simulink model "sltank2"  (R2018b)
settings: Solver=ode23  StartTime=0  StopTime=10000  MaxStep=0.2  RelTol=1e-3  AbsTol=1e-6
PreLoadFcn:
  | tank2=readfis('tank2');
libraries: fuzblock x1, simulink x1
CloseFcn:
  | clear tank2
settings Model: FPTRunName=Active  ExtModeTrigMode=oneshot  ExtModeArmWhenConnect=off  ExtModeAutoUpdateStatusClock=off  Creator=The MathWorks, Inc.  LastModifiedBy=The MathWorks, Inc.
settings SolverCC: AutoScaleAbsTol=off
settings DataIOCC: SaveFormat=Array  SaveOutput=off  SaveTime=off
settings OptimizationCC: BlockReduction=off  BooleanDataType=off  ExpressionDepthLimit=2147483647  InitFltsAndDblsToZero=on  LifeSpan=inf
settings DebuggingCC: SaveWithParameterizedLinksMsg=none  UnderspecifiedInitializationDetection=Classic  MergeDetectMultiDrivingBlocksExec=none  SignalResolutionControl=TryResolveAllWithWarning  MultiTaskDSMMsg=warning  MultiTaskCondExecSysMsg=none  FcnCallInpInsideContextMsg=warning  StateNameClashWarn=warning  LibraryContextMissingDiagnostic=none  SFUnexpectedBacktrackingDiag=warning  SFNoUnconditionalDefaultTransitionDiag=warning  SFExecutionAtInitializationDiag=none
settings HardwareCC: ProdBitPerPointer=32  ProdBitPerSizeT=32  ProdBitPerPtrDiffT=32  ProdLargestAtomicFloat=None  ProdIntDivRoundTo=Undefined  ProdEndianess=Unspecified  ProdWordSize=32  ProdHWDeviceType=32-bit Generic  TargetUnknown=on
settings ModelReferenceCC: PropagateSignalLabelsOutOfModel=off
settings SFSimCC: SimUseLocalCustomCode=off
settings RTWCC: RTWUseLocalCustomCode=off
settings CodeAppCC: StateflowObjectComments=on
settings GRTTargetCC: TargetFcnLib=ansi_tfl_tmw.mat  TargetLangStandard=C89/C90 (ANSI)  GeneratePreprocessorConditionals=Disable all  CombineOutputUpdateFcns=off  GRTInterface=on
settings ConfigComp: CovMetricSettings=dw  CovHtmlReporting=on  CovSaveCumulativeToWorkspaceVar=on  CovSaveSingleToWorkspaceVar=on  CovExternalEMLEnable=off

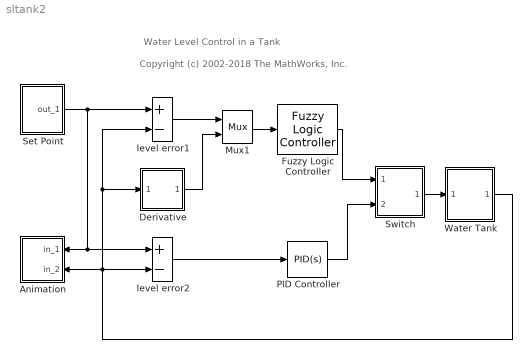
== system sltank2 ==
  note: Copyright (c) 2002-2018 The MathWorks, Inc.
  note: Water Level Control in a Tank
  Animation : Subsystem
  Derivative : Subsystem
  Fuzzy Logic Controller : fuzblock/Fuzzy Logic  Controller  FIS=tank2  OutputSampleNumber=101  DataType=double  FuzzifiedInputs=off  RuleFiringStrengths=off  RuleOutputs=off  AggregatedOutputs=off  SimulateUsing=Interpreted execution  OutOfRangeInputValueMessage=warning  NoRuleFiredMessage=warning  EmptyOutputFuzzySetMessage=warning
  Mux1 : Mux  Inputs=2
  PID Controller : simulink/Continuous/PID Controller  Controller=PID  Form=Parallel  TimeDomain=Continuous-time  SampleTime=1  IntegratorMethod=Forward Euler  FilterMethod=Forward Euler  ControllerParametersSource=internal  P=2  I=0  D=1  UseFilter=on  N=100  TunerSelectOption=Transfer Function Based (PID Tuner App)  InitialConditionSource=internal  InitialConditionForIntegrator=0  InitialConditionForFilter=0  DifferentiatorICPrevScaledInput=0  ExternalReset=none  TrackingMode=off  Kt=1  LimitOutput=off  UpperSaturationLimit=inf  LowerSaturationLimit=-inf  LinearizeAsGain=off  AntiWindupMode=none  Kb=1  POutMin=[]  POutMax=[]  IOutMin=[]  IOutMax=[]  DOutMin=[]  DOutMax=[]  NOutMin=[]  NOutMax=[]  SumOutMin=[]  SumOutMax=[]  SaturationOutMin=[]  SaturationOutMax=[]  PParamMin=[]  PParamMax=[]  IParamMin=[]  IParamMax=[]  DParamMin=[]  DParamMax=[]  NParamMin=[]  NParamMax=[]  KbParamMin=[]  KbParamMax=[]  KtParamMin=[]  KtParamMax=[]  KbOutMin=[]  KbOutMax=[]  KtOutMin=[]  KtOutMax=[]  IntegratorOutMin=[]  IntegratorOutMax=[]  FilterOutMin=[]  FilterOutMax=[]  SumI1OutMin=[]  SumI1OutMax=[]  SumI2OutMin=[]  SumI2OutMax=[]  SumI3OutMin=[]  SumI3OutMax=[]  SumI4OutMin=[]  SumI4OutMax=[]  SumDOutMin=[]  SumDOutMax=[]  DifferentiatorOutMin=[]  DifferentiatorOutMax=[]  FilterDiffOutCoefMin=[]  FilterDiffOutCoefMax=[]  ReciprocalOutMin=[]  ReciprocalOutMax=[]  SumDenOutMin=[]  SumDenOutMax=[]  SumNumOutMin=[]  SumNumOutMax=[]  DivideOutMin=[]  DivideOutMax=[]  IntegratorContinuousStateAttributes=''  IntegratorStateMustResolveToSignalObject=off  IntegratorRTWStateStorageClass=Auto  FilterContinuousStateAttributes=''  FilterStateMustResolveToSignalObject=off  FilterRTWStateStorageClass=Auto  ParallelPVariant=InternalParameters  IdealPVariant=Disabled  IVariant=InternalParameters  DVariant=InternalParameters  IntegratorVariant=Continuous  SatVariant=Disabled  AWVariant=Passthrough  PCopyVariant=Disabled  TRVariant=Disabled  FdbkBlocksVariant=Forward  IdealPFdbkVariant=Disabled  SatFdbkVariant=Disabled  DerivativeFilterVariant=ContFilter  NVariant=InternalParameters  NCopyVariant=Disabled  FilterICVariant=InternalICsFilter  IntegratorICVariant=InternalICs  ExternalResetVariant=Disabled  TRSumVariant=Passthrough  SumFdbkVariant=Disabled  SumVariant=Sum_PID
  Set Point : Subsystem
  Switch : Subsystem
  Water Tank : Subsystem
  level error1 : Sum  Inputs=+-  SaturateOnIntegerOverflow=on  InputSameDT=on  OutDataTypeStr=Inherit: Same as first input
  level error2 : Sum  Inputs=+-  SaturateOnIntegerOverflow=on  InputSameDT=on  OutDataTypeStr=Inherit: Same as first input
  wires:
  Water Tank/1(out_1) -> Derivative/1(in_1), level error1/2, Animation/2(in_2), level error2/2
  level error2/1 -> PID Controller/1
  Derivative/1(out_1) -> Mux1/2
  Set Point/1(out_1) -> level error2/1, Animation/1(in_1), level error1/1
  PID Controller/1 -> Switch/2(in_2)
  Fuzzy Logic Controller/1 -> Switch/1(in_1)
  Switch/1(out_1) -> Water Tank/1(in_1)
  level error1/1 -> Mux1/1
  Mux1/1 -> Fuzzy Logic Controller/1

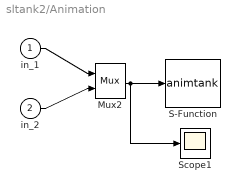
== system sltank2/Animation ==
  in_1 : Inport
  in_2 : Inport  Port=2
  Mux2 : Mux  Inputs=2
  S-Function : S-Function  FunctionName=animtank  Parameters=1  SFunctionDeploymentMode=off  EnableBusSupport=off
  Scope1 : Scope
  wires:
  in_2/1 -> Mux2/2
  in_1/1 -> Mux2/1
  Mux2/1 -> S-Function/1, Scope1/1

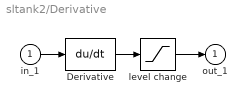
== system sltank2/Derivative ==
  in_1 : Inport
  Derivative : Derivative
  level change : Saturate  UpperLimit=0.1  LowerLimit=-0.1
  out_1 : Outport
  wires:
  in_1/1 -> Derivative/1
  level change/1 -> out_1/1
  Derivative/1 -> level change/1

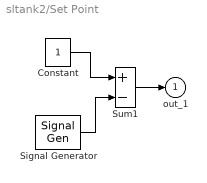
== system sltank2/Set Point ==
  Constant : Constant
  Signal Generator : SignalGenerator  WaveForm=square  Amplitude=0.500000  Frequency=0.250000  Units=rad/sec
  Sum1 : Sum  Inputs=+-  SaturateOnIntegerOverflow=on  InputSameDT=on  OutDataTypeStr=Inherit: Same as first input
  out_1 : Outport
  wires:
  Sum1/1 -> out_1/1
  Constant/1 -> Sum1/1
  Signal Generator/1 -> Sum1/2

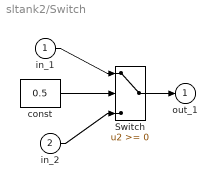
== system sltank2/Switch ==
  in_1 : Inport
  in_2 : Inport  Port=2
  Switch : Switch  SaturateOnIntegerOverflow=on  InputSameDT=on
  const : Constant  Value=0.5
  out_1 : Outport
  wires:
  in_2/1 -> Switch/3
  Switch/1 -> out_1/1
  in_1/1 -> Switch/1
  const/1 -> Switch/2

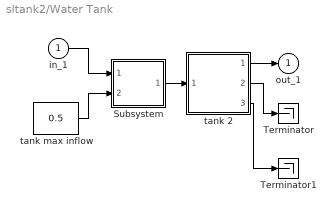
== system sltank2/Water Tank ==
  in_1 : Inport
  Subsystem : Subsystem  mask(Valve){InitialPosition=0}
      mask prompts: InitialPosition "Initial position [0=closed 1=open]:"
      mask help: Valve
      mask Display: disp('VALVE')
  Terminator : Terminator
  Terminator1 : Terminator
  tank 2 : Subsystem  mask(Water tank){ht=2, area=1, outletArea=0.05, overflowLimit=0, initialHt=0.5}
      mask prompts: ht "Height of tank (m):"; area "Bottom area (m^2):"; outletArea "Out pipe crossection (m^2):"; overflowLimit "Overflow sensor distance from top (m):"; initialHt "Initial level height (m):"
      mask help: Cylindrical water tank with overflow signal
      mask Display: disp('WATER\nTANK')
  tank max inflow : Constant  Value=0.5
  out_1 : Outport
  wires:
  Subsystem/1(out flow) -> tank 2/1(flow in)
  tank max inflow/1 -> Subsystem/2(source flow)
  tank 2/1(water level) -> out_1/1
  in_1/1 -> Subsystem/1(control)
  tank 2/2(flow out) -> Terminator/1
  tank 2/3(overflow flag) -> Terminator1/1

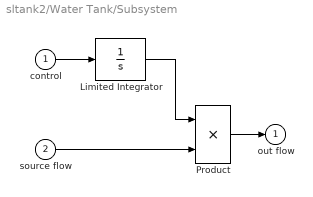
== system sltank2/Water Tank/Subsystem ==
  control : Inport
  source flow : Inport  Port=2
  Limited Integrator : Integrator  InitialCondition=InitialPosition  LimitOutput=on  UpperSaturationLimit=1  LowerSaturationLimit=0
  Product : Product  SaturateOnIntegerOverflow=on  RndMeth=Zero  InputSameDT=on  OutDataTypeStr=Inherit: Same as first input
  out flow : Outport
  wires:
  source flow/1 -> Product/2
  Product/1 -> out flow/1
  control/1 -> Limited Integrator/1
  Limited Integrator/1 -> Product/1

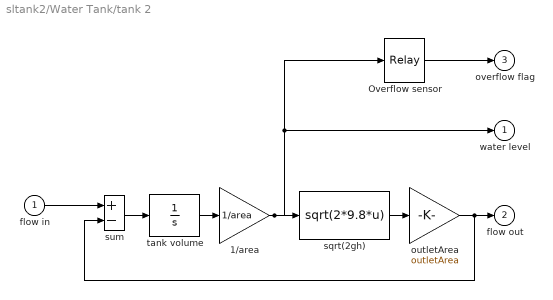
== system sltank2/Water Tank/tank 2 ==
  flow in : Inport
  1/area : Gain  Gain=1/area  SaturateOnIntegerOverflow=on  OutDataTypeStr=Inherit: Same as input  ParamDataTypeStr=Inherit: Same as input
  Overflow sensor : Relay  OnSwitchValue=ht - overflowLimit  OffSwitchValue=ht - overflowLimit
  outletArea : Gain  Gain=outletArea  SaturateOnIntegerOverflow=on  OutDataTypeStr=Inherit: Same as input  ParamDataTypeStr=Inherit: Same as input
  sqrt(2gh) : Fcn  Expr=sqrt(2*9.8*u)
  sum : Sum  Inputs=+-  SaturateOnIntegerOverflow=on  InputSameDT=on  OutDataTypeStr=Inherit: Same as first input
  tank volume : Integrator  InitialCondition=initialHt * area  LimitOutput=on  UpperSaturationLimit=ht * area  LowerSaturationLimit=0
  water level : Outport
  flow out : Outport  Port=2
  overflow flag : Outport  Port=3
  wires:
  1/area/1 -> water level/1, Overflow sensor/1, sqrt(2gh)/1
  outletArea/1 -> sum/2, flow out/1
  sqrt(2gh)/1 -> outletArea/1
  tank volume/1 -> 1/area/1
  Overflow sensor/1 -> overflow flag/1
  flow in/1 -> sum/1
  sum/1 -> tank volume/1
